simulink model "pid_controller"  (R2025b)
settings: Solver=VariableStepAuto  StartTime=0.0  StopTime=10.0  RelTol=1e-3
values from neighbouring files (symbols this model uses):
  Kd = 10.0    [pid_constants.sldd]
  Ki = 200.0    [pid_constants.sldd]
  Kp = 100.0    [pid_constants.sldd]
settings Model: DataDictionary=pid_constants.sldd  Creator=mammadoo  LastModifiedBy=mammadoo

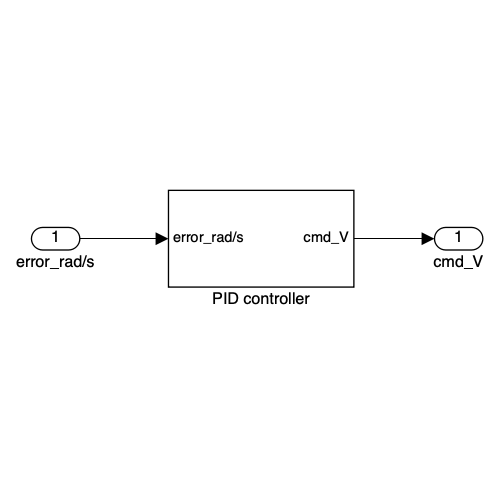
[thumbnail: Simulink's stored preview of the top-level diagram]
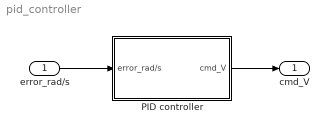
== system pid_controller ==
  error_rad/s : Inport
  PID controller : Subsystem
  cmd_V : Outport
  wires:
  error_rad/s/1 -> PID controller/1(error_rad/s)
  PID controller/1(cmd_V) -> cmd_V/1

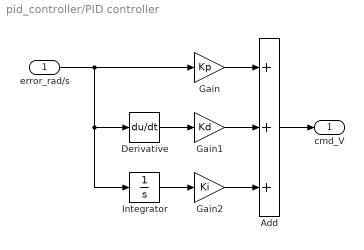
== system pid_controller/PID controller ==
  error_rad/s : Inport
  Add : Sum  Inputs=+++
  Derivative : Derivative
  Gain : Gain  Gain=Kp
  Gain1 : Gain  Gain=Kd
  Gain2 : Gain  Gain=Ki
  Integrator : Integrator
  cmd_V : Outport
  wires:
  Add/1 -> cmd_V/1
  Gain1/1 -> Add/2
  Gain2/1 -> Add/3
  Gain/1 -> Add/1
  error_rad/s/1 -> Integrator/1, Derivative/1, Gain/1
  Integrator/1 -> Gain2/1
  Derivative/1 -> Gain1/1
